simulink model "sl_subsys_overview"  (Simulink 6.0)
settings: Solver=ode45  StartTime=0.0  StopTime=10.0  RelTol=1e-3
settings Model: CovMetricSettings=d  Creator=The MathWorks Inc.  LastModifiedBy=batserve  ExtModeAutoUpdateStatusClock=off  BufferReuse=off  ProdHWDeviceType=Specified
settings DataIOCC: SignalLoggingName=logsOut
settings OptimizationCC: BlockReduction=off  BooleanDataType=off  OptimizeBlockIOStorage=off  BufferReuse=off  ExpressionFolding=off  LocalBlockOutputs=off
settings DebuggingCC: CheckExecutionContextPreStartOutputMsg=on  CheckExecutionContextRuntimeOutputMsg=on  SolverPrmCheckMsg=none
settings HardwareCC: ProdHWDeviceType=Specified
settings ModelReferenceCC: UpdateModelReferenceTargets=IfOutOfDate

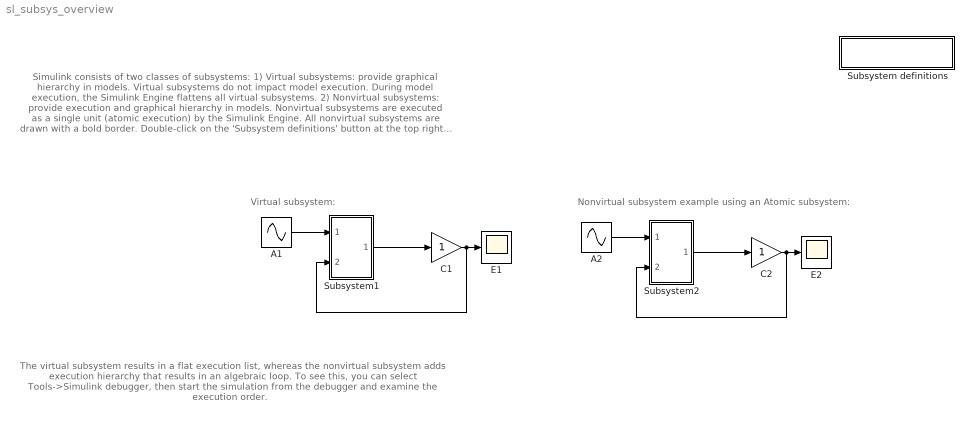
== system sl_subsys_overview ==
  note: Simulink consists of two classes of subsystems:
      |
      | 1) Virtual subsystems: provide graphical hierarchy in models. Virtual
      |    subsystems do not impact model execution. During model execution, the
      |    Simulink Engine flattens all virtual subsystems.
      |
      | 2) Nonvirtual subsystems: provide execution and graphical hierarchy in models.
      |    Nonvirtual subsystems are executed as a single unit (atomic execution) by
      |    the Simulink Engine. All nonvirtual subsystems are drawn with a bold border.
      |
      | Double-click on the 'Subsystem definitions' button at the top right for more details.
  note: Nonvirtual subsystem example using an Atomic subsystem:
  note: Virtual subsystem:
  note: The virtual subsystem results in a flat execution list, whereas the nonvirtual subsystem
      | adds execution hierarchy that results in an algebraic loop. To see this, you can select
      | Tools->Simulink debugger, then start the simulation from the debugger and examine
      |  the execution order.
  " Subsystem definitions" : Subsystem  PropExecContextAcrossSSBoundary=on
      settings: OpenFcn=helpview([matlabroot,'/toolbox/simulink/simdemos/sl_subsys_definitions.html']);
      mask Display: disp('Subsystem\ndefinitions')
  A1 : Sin  SampleTime=0
  A2 : Sin  SampleTime=0
  C1 : Gain  SaturateOnIntegerOverflow=on
  C2 : Gain  SaturateOnIntegerOverflow=on
  E1 : Scope
  E2 : Scope
  Subsystem1 : Subsystem  PropExecContextAcrossSSBoundary=on
  Subsystem2 : Subsystem  TreatAsAtomicUnit=on  PropExecContextAcrossSSBoundary=on
  wires:
  A1/1 -> Subsystem1/1(In1)
  Subsystem1/1(Out1) -> C1/1
  C1/1 -> Subsystem1/2(In2), E1/1
  A2/1 -> Subsystem2/1(In1)
  Subsystem2/1(Out1) -> C2/1
  C2/1 -> E2/1, Subsystem2/2(In2)

== system sl_subsys_overview/ Subsystem definitions ==

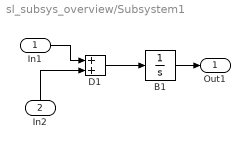
== system sl_subsys_overview/Subsystem1 ==
  In1 : Inport  Port=1  LatchInput=off
  In2 : Inport  Orientation=up  Port=2  LatchInput=off
  B1 : Integrator
  D1 : Sum  SaturateOnIntegerOverflow=on  InputSameDT=on
  Out1 : Outport
  wires:
  In1/1 -> D1/1
  B1/1 -> Out1/1
  In2/1 -> D1/2
  D1/1 -> B1/1

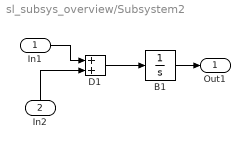
== system sl_subsys_overview/Subsystem2 ==
  In1 : Inport  Port=1  LatchInput=off
  In2 : Inport  Orientation=up  Port=2  LatchInput=off
  B1 : Integrator
  D1 : Sum  SaturateOnIntegerOverflow=on  InputSameDT=on
  Out1 : Outport
  wires:
  D1/1 -> B1/1
  In2/1 -> D1/2
  B1/1 -> Out1/1
  In1/1 -> D1/1
